simulink model "Test_CP_global"  (R2020a)
settings: configuration reference "Configuration" (kept outside this file)
undefined symbols (not defined in the file): ddParam, p1, ps, ps_p1
settings Model: DataDictionary=MyParams.sldd  OrderedModelArguments=off  Creator=toma  LastModifiedBy=toma
settings ConfigSetRef: SourceName=Configuration

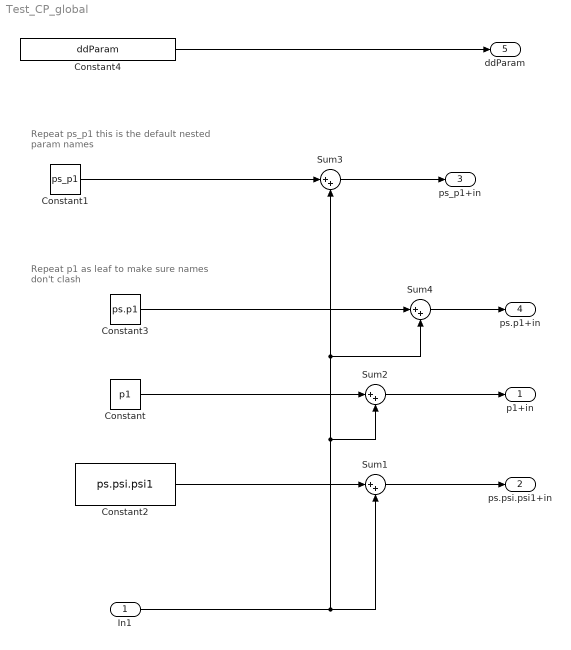
== system Test_CP_global ==
  note: Repeat p1 as leaf to make
      | sure names don't clash
  note: Repeat ps_p1 this is the
      | default nested param names
  In1 : Inport  OutDataTypeStr=double  PortDimensions=1  SampleTime=[0.20000000000000001,0]
  Constant : Constant  Value=p1
  Constant1 : Constant  Value=ps_p1
  Constant2 : Constant  Value=ps.psi.psi1
  Constant3 : Constant  Value=ps.p1
  Constant4 : Constant  Value=ddParam
  Sum{1..4} (4 alike) : Sum  Inputs=|++
  p1+in : Outport  OutDataTypeStr=double  PortDimensions=[2 2]  SampleTime=[0.20000000000000001,0]
  ps.psi.psi1+in : Outport  Port=2  OutDataTypeStr=double  PortDimensions=1  SampleTime=[0.20000000000000001,0]
  ps_p1+in : Outport  Port=3
  ps.p1+in : Outport  Port=4
  ddParam : Outport  Port=5
  wires:
  Sum1/1 -> ps.psi.psi1+in/1
  In1/1 -> Sum2/2, Sum3/2, Sum4/2, Sum1/2
  Constant/1 -> Sum2/1
  Constant2/1 -> Sum1/1
  Sum2/1 -> p1+in/1
  Sum3/1 -> ps_p1+in/1
  Constant1/1 -> Sum3/1
  Constant3/1 -> Sum4/1
  Sum4/1 -> ps.p1+in/1
  Constant4/1 -> ddParam/1
